simulink model "rlc_simulink"  (R2020a)
settings: Solver=FixedStepAuto  StartTime=0.0  StopTime=1000  FixedStep=0.001  RelTol=1e-3
settings Model: Creator=PC12  LastModifiedBy=PC12

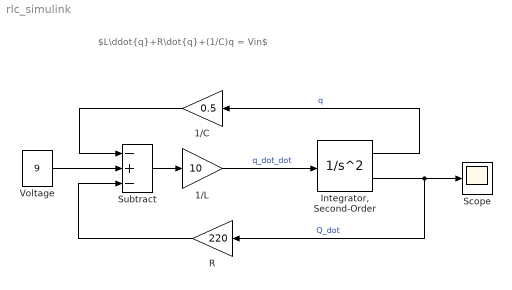
== system rlc_simulink ==
  note: $L\ddot{q}+R\dot{q}+(1/C)q = Vin$
  1/C : Gain  Gain=0.5
  1/L : Gain  Gain=10
  "Integrator, Second-Order" : SecondOrderIntegrator
  R : Gain  Gain=220
  Scope : Scope
  Subtract : Sum  Inputs=-+-
  Voltage : Constant  Value=9
  wires:
  Voltage/1 -> Subtract/2
  R/1 -> Subtract/3
  1/C/1 -> Subtract/1
  Subtract/1 -> 1/L/1
  "Integrator, Second-Order"/2 -> R/1, Scope/1  "Q_dot"
  "Integrator, Second-Order"/1 -> 1/C/1  "q"
  1/L/1 -> "Integrator, Second-Order"/1  "q_dot_dot"
